simulink model "boucle_ouverte_corrige"  (R2018b)
settings: Solver=VariableStepAuto  StartTime=0.0  StopTime=60  RelTol=1e-3
undefined symbols (not defined in the file): to
settings Model: Creator=12108993  LastModifiedBy=12108993

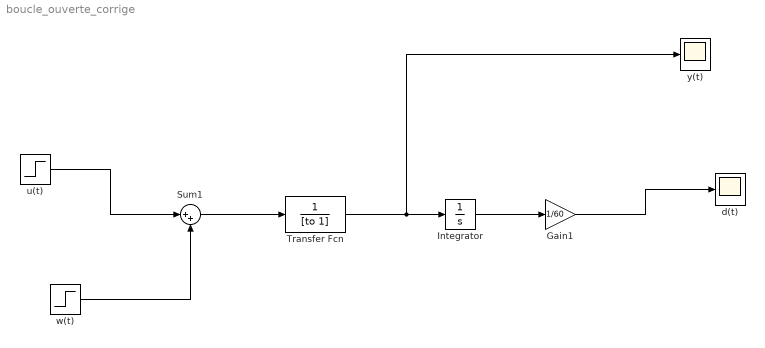
== system boucle_ouverte_corrige ==
  Gain1 : Gain  Gain=1/60
  Integrator : Integrator  UpperSaturationLimit=t  LowerSaturationLimit=0
  Sum1 : Sum  Inputs=|++
  Transfer Fcn : TransferFcn  Denominator=[to 1]
  "d(t) " : Scope
  "u(t) " : Step  Time=10  Before=15  After=0  SampleTime=0
  "w(t) " : Step  Time=20  After=10  SampleTime=0
  y(t) : Scope
  wires:
  Integrator/1 -> Gain1/1
  "u(t) "/1 -> Sum1/1
  "w(t) "/1 -> Sum1/2
  Sum1/1 -> Transfer Fcn/1
  Transfer Fcn/1 -> y(t)/1, Integrator/1
  Gain1/1 -> "d(t) "/1
